simulink model "Robot_control"  (R2017a)
settings: Solver=VariableStepAuto  StartTime=0.0  StopTime=10.0  RelTol=1e-3
values from neighbouring files (symbols this model uses):
  hd = trajectory(1:2)    [control.m]    (also in traj_gen.m = [R * cos( w_d*t ))
undefined symbols (not defined in the file or in its folder): control, error_plot, robot_20, traj_gen, X2h
settings Model: Creator=rramachand2017  LastModifiedBy=rramachand2017

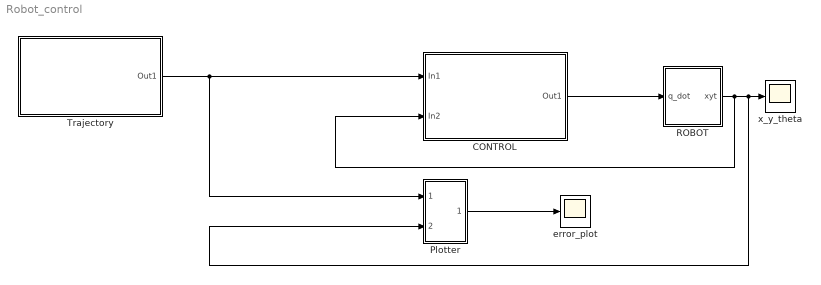
== system Robot_control ==
  CONTROL : Subsystem
  Plotter : Subsystem
  "ROBOT " : Subsystem
  Trajectory : Subsystem
  error_plot : Scope
  x_y_theta : Scope
  wires:
  "ROBOT "/1(xyt) -> CONTROL/2(In2), Plotter/2(In2), x_y_theta/1
  Plotter/1(Out1) -> error_plot/1
  Trajectory/1(Out1) -> Plotter/1(In1), CONTROL/1(In1)
  CONTROL/1(Out1) -> "ROBOT "/1(q_dot)

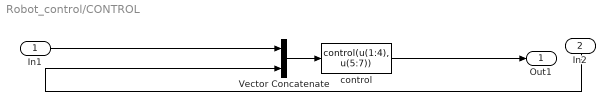
== system Robot_control/CONTROL ==
  In1 : Inport
  In2 : Inport  Port=2
  Vector Concatenate : Concatenate
  control : MATLABFcn  MATLABFcn="control(u(1:4),  u(5:7))"  OutputDimensions=2
  Out1 : Outport
  wires:
  Vector Concatenate/1 -> control/1
  In1/1 -> Vector Concatenate/1
  In2/1 -> Vector Concatenate/2
  control/1 -> Out1/1

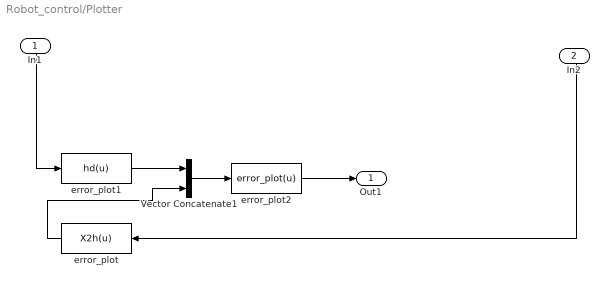
== system Robot_control/Plotter ==
  In1 : Inport
  In2 : Inport  Port=2
  Vector Concatenate1 : Concatenate
  error_plot : MATLABFcn  MATLABFcn=X2h(u)  OutputDimensions=2
  error_plot1 : MATLABFcn  MATLABFcn=hd(u)  OutputDimensions=2
  error_plot2 : MATLABFcn  MATLABFcn=error_plot(u)  OutputDimensions=1
  Out1 : Outport
  wires:
  In1/1 -> error_plot1/1
  In2/1 -> error_plot/1
  error_plot2/1 -> Out1/1
  error_plot1/1 -> Vector Concatenate1/1
  Vector Concatenate1/1 -> error_plot2/1
  error_plot/1 -> Vector Concatenate1/2

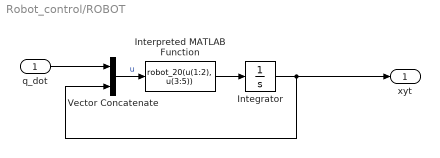
== system Robot_control/ROBOT  ==
  q_dot : Inport
  Integrator : Integrator  InitialCondition=[2.3;0;pi]
  Interpreted MATLAB Function : MATLABFcn  MATLABFcn=robot_20(u(1:2), u(3:5))  OutputDimensions=3
  Vector Concatenate : Concatenate
  xyt : Outport
  wires:
  Integrator/1 -> xyt/1, Vector Concatenate/2
  Vector Concatenate/1 -> Interpreted MATLAB Function/1  "u"
  Interpreted MATLAB Function/1 -> Integrator/1
  q_dot/1 -> Vector Concatenate/1

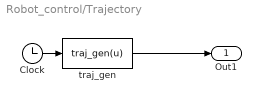
== system Robot_control/Trajectory ==
  Clock : Clock
  traj_gen : MATLABFcn  MATLABFcn=traj_gen(u)  OutputDimensions=4
  Out1 : Outport
  wires:
  Clock/1 -> traj_gen/1
  traj_gen/1 -> Out1/1
